simulink model "PruebasMRR"  (R2023b)
settings: Solver=VariableStepAuto  StartTime=0.0  StopTime=10.0  RelTol=1e-3
libraries: canmsglib x1, arduinolib x1
settings Model: Creator=merce  LastModifiedBy=merce

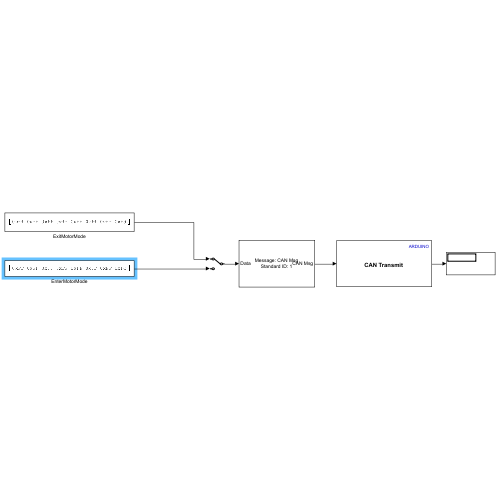
[thumbnail: Simulink's stored preview of the top-level diagram]
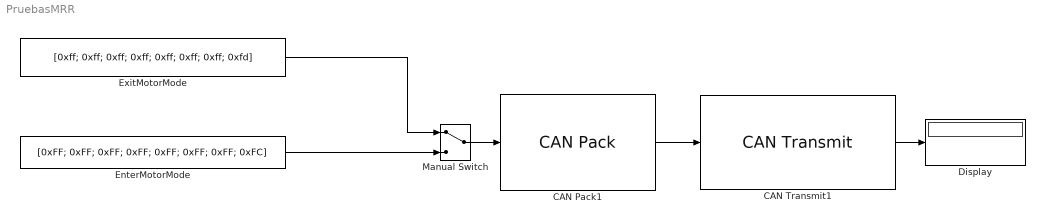
== system PruebasMRR ==
  CAN Pack1 : canmsglib/CAN Pack  MsgList=(none)  MsgName=CAN Msg  MsgIDType=Standard (11-bit identifier)  MsgIdentifier=1  MsgLength=8  Remote=off  ApplyMinMax=off  BusOutput=on  SignalInfo={ 'position', '8', '16', 'BE', 'signed', 'Standard', '0', '1', '-95.5', '-95.5', '95.5'; 'velocity', '28', '12', 'BE', 'signed', 'Standard', '0', '1', '-45', '-45', '45'; 'kp', '32', '12', 'BE', 'unsigned', 'Standard', '0', '1', '0', '0', '500'; 'kd', '52', '12', 'BE', 'unsigned', 'Standard', '0', '1', '0', '0', '5'; 'torque', '56', '12', 'BE', 'signed', 'Standard', '0', '1', '-18', '-18', '18' }
      settings: LibrarySourceBlock=embeddedtargetslib/Host Communication/CAN Pack  DataFormat=raw data
  CAN Transmit1 : arduinolib/CAN Transmit  inputDataType=CAN Msg  BlockingMode_=on  BlockTimeout_=1  outputStatus=on  identifierType=Standard (11-bit identifier)  messageId=100  msgLength=8  remoteFrame=off
  Display : Display
  EnterMotorMode : Constant  Value=|  OutDataTypeStr=uint8
      | [0xFF; 0xFF; 0xFF; 0xFF; 0xFF;
      | 0xFF;
      | 0xFF;
      | 0xFC]
  ExitMotorMode : Constant  Value=|  OutDataTypeStr=uint8
      | [0xff; 0xff; 0xff; 0xff; 0xff;
      | 0xff;
      | 0xff;
      | 0xfd]
  Manual Switch : ManualSwitch
  wires:
  EnterMotorMode/1 -> Manual Switch/2
  Manual Switch/1 -> CAN Pack1/1
  CAN Transmit1/1 -> Display/1
  CAN Pack1/1 -> CAN Transmit1/1
  ExitMotorMode/1 -> Manual Switch/1
